simulink model "MVS_Static_Trigger_Two_Layers_RA"  (R2024a)
settings: Solver=ode5  StartTime=0.0  StopTime=180  FixedStep=0.01  RelTol=1e-3
(part 1 of 4)
settings Model: Creator=yfeih  LastModifiedBy=Lenovo
settings OptimizationCC: ReuseModelBlockBuffer=off
settings RTWCC: GPUComputeCapability=3.5

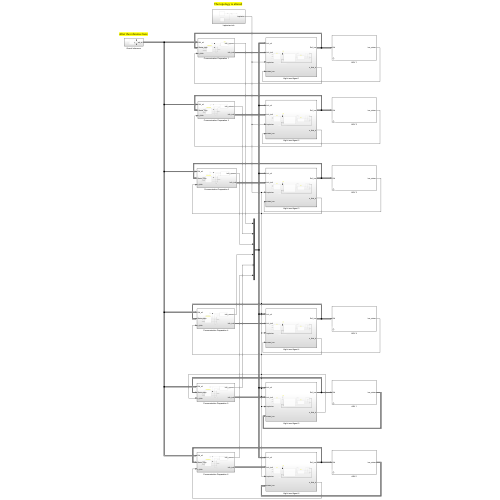
[thumbnail: Simulink's stored preview of the top-level diagram]
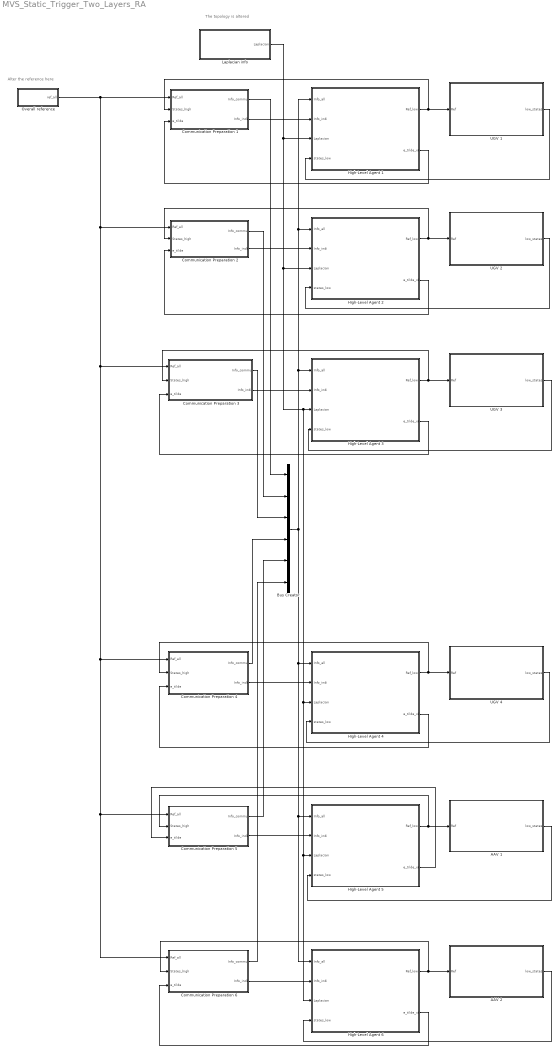
== system MVS_Static_Trigger_Two_Layers_RA ==
  note: Alter the reference here
  note: The topology is altered
  AAV 1 : Subsystem  mask{ini_pos=[-20;-20;0]}
      mask prompts: ini_pos "initial_pos"
      mask TypeOptions ini_pos: x_int/InitialCondition
      mask DialogControl ParameterGroupVar Prompt: 参数
  AAV 2 : Subsystem  mask{ini_pos=[-26;-30;0]}
      mask prompts: ini_pos "initial_pos"
      mask TypeOptions ini_pos: x_int/InitialCondition
      mask DialogControl ParameterGroupVar Prompt: 参数
  Bus Creator : BusCreator  Inputs=6
  Communication Preparation 1 : Subsystem
  Communication Preparation 2 : Subsystem
  Communication Preparation 3 : Subsystem
  Communication Preparation 4 : Subsystem
  Communication Preparation 5 : Subsystem
  Communication Preparation 6 : Subsystem
  High-Level Agent 1 : Subsystem
  High-Level Agent 2 : Subsystem
  High-Level Agent 3 : Subsystem
  High-Level Agent 4 : Subsystem
  High-Level Agent 5 : Subsystem
  High-Level Agent 6 : Subsystem
  Laplacian info : Subsystem
  Overall reference : Subsystem
  UGV 1 : Subsystem  mask{ini_int=[-25;-20;0], ini_memo=[-25;-20;0]}
      mask prompts: ini_int "initial_pos"; ini_memo "pos_memory"
      mask TypeOptions ini_int: pos_int/InitialCondition
      mask TypeOptions ini_memo: pos_memo/InitialCondition
      mask DialogControl ParameterGroupVar Prompt: 参数
  UGV 2 : Subsystem  mask{ini_int=[-35;-35;0], ini_memo=[-35;-35;0]}
      mask prompts: ini_int "initial_pos"; ini_memo "pos_memory"
      mask TypeOptions ini_int: pos_int/InitialCondition
      mask TypeOptions ini_memo: pos_memo/InitialCondition
      mask DialogControl ParameterGroupVar Prompt: 参数
  UGV 3 : Subsystem  mask{ini_int=[-50;-30;pi/4], ini_memo=[-50;-30;pi/4]}
      mask prompts: ini_int "initial_pos"; ini_memo "pos_memory"
      mask TypeOptions ini_int: pos_int/InitialCondition
      mask TypeOptions ini_memo: pos_memory/InitialCondition
      mask DialogControl ParameterGroupVar Prompt: 参数
  UGV 4 : Subsystem  mask{ini_int=[-50;-45;pi/4], ini_memo=[-50;-45;pi/4]}
      mask prompts: ini_int "initial_pos"; ini_memo "pos_memory"
      mask TypeOptions ini_int: pos_int/InitialCondition
      mask TypeOptions ini_memo: pos_memory/InitialCondition
      mask DialogControl ParameterGroupVar Prompt: 参数
  wires:
  Communication Preparation 1/1(Info_commu) -> Bus Creator/1
  Communication Preparation 1/2(Info_indi) -> High-Level Agent 1/2(Info_indi)
  High-Level Agent 1/1(Ref_low) -> UGV 1/1(Ref), Communication Preparation 1/2(States_high)
  High-Level Agent 3/1(Ref_low) -> UGV 3/1(Ref), Communication Preparation 3/2(States_high)
  Communication Preparation 3/2(Info_indi) -> High-Level Agent 3/2(Info_indi)
  Communication Preparation 3/1(Info_commu) -> Bus Creator/3
  Laplacian info/1(Laplacian) -> High-Level Agent 6/3(Laplacian), High-Level Agent 5/3(Laplacian), High-Level Agent 4/3(Laplacian), High-Level Agent 3/3(Laplacian), High-Level Agent 2/3(Laplacian), High-Level Agent 1/3(Laplacian)
  Communication Preparation 2/1(Info_commu) -> Bus Creator/2
  Communication Preparation 2/2(Info_indi) -> High-Level Agent 2/2(Info_indi)
  High-Level Agent 2/1(Ref_low) -> UGV 2/1(Ref), Communication Preparation 2/2(States_high)
  High-Level Agent 4/1(Ref_low) -> UGV 4/1(Ref), Communication Preparation 4/2(States_high)
  Communication Preparation 4/2(Info_indi) -> High-Level Agent 4/2(Info_indi)
  Communication Preparation 4/1(Info_commu) -> Bus Creator/4
  High-Level Agent 5/1(Ref_low) -> AAV 1/1(Ref), Communication Preparation 5/2(States_high)
  Communication Preparation 5/1(Info_commu) -> Bus Creator/5
  Communication Preparation 5/2(Info_indi) -> High-Level Agent 5/2(Info_indi)
  Bus Creator/1 -> High-Level Agent 6/1(Info_all), High-Level Agent 5/1(Info_all), High-Level Agent 4/1(Info_all), High-Level Agent 3/1(Info_all), High-Level Agent 2/1(Info_all), High-Level Agent 1/1(Info_all)
  High-Level Agent 6/1(Ref_low) -> AAV 2/1(Ref), Communication Preparation 6/2(States_high)
  Communication Preparation 6/1(Info_commu) -> Bus Creator/6
  Communication Preparation 6/2(Info_indi) -> High-Level Agent 6/2(Info_indi)
  Overall reference/1(ref_all) -> Communication Preparation 6/1(Ref_all), Communication Preparation 5/1(Ref_all), Communication Preparation 4/1(Ref_all), Communication Preparation 3/1(Ref_all), Communication Preparation 2/1(Ref_all), Communication Preparation 1/1(Ref_all)
  High-Level Agent 1/2(e_tilde_xi) -> Communication Preparation 1/3(e_tilde)
  High-Level Agent 2/2(e_tilde_xi) -> Communication Preparation 2/3(e_tilde)
  High-Level Agent 3/2(e_tilde_xi) -> Communication Preparation 3/3(e_tilde)
  High-Level Agent 4/2(e_tilde_xi) -> Communication Preparation 4/3(e_tilde)
  High-Level Agent 6/2(e_tilde_xi) -> Communication Preparation 6/3(e_tilde)
  High-Level Agent 5/2(e_tilde_xi) -> Communication Preparation 5/3(e_tilde)
  UGV 1/1(low_states) -> High-Level Agent 1/4(states_low)
  UGV 2/1(low_states) -> High-Level Agent 2/4(states_low)
  UGV 4/1(low_states) -> High-Level Agent 4/4(states_low)
  AAV 1/1(low_states) -> High-Level Agent 5/4(states_low)
  AAV 2/1(low_states) -> High-Level Agent 6/4(states_low)
  UGV 3/1(low_states) -> High-Level Agent 3/4(states_low)

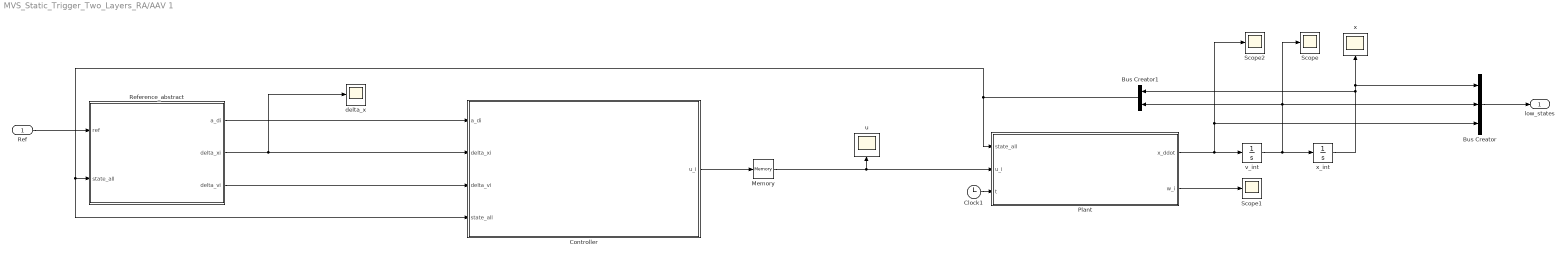
== system MVS_Static_Trigger_Two_Layers_RA/AAV 1 ==
  Ref : Inport
  Bus Creator : BusCreator  Inputs=3
  Bus Creator1 : BusCreator  Inputs=2
  Clock1 : Clock
  Controller : Subsystem
  Memory : Memory  InitialCondition=[0;0;0]
  Plant : MATLAB Function  TreatAsAtomicUnit=on
  Reference_abstract : MATLAB Function  TreatAsAtomicUnit=on
  Scope : Scope
  Scope1 : Scope
  Scope2 : Scope
  delta_x : Scope
  u : Scope
  v_int : Integrator  InitialCondition=[0;0;0]  ContinuousStateAttributes='vel'
  x : Scope
  x_int : Integrator  InitialCondition=ini_pos  ContinuousStateAttributes='pos'
  low_states : Outport
  wires:
  Plant/2(w_i) -> Scope1/1
  Clock1/1 -> Plant/3(t)
  Reference_abstract/1(a_di) -> Controller/1(a_di)
  Controller/1(u_i) -> Memory/1
  Memory/1 -> u/1, Plant/2(u_i)
  Reference_abstract/2(delta_xi) -> delta_x/1, Controller/2(delta_xi)
  Ref/1 -> Reference_abstract/1(ref)
  v_int/1 -> Bus Creator1/2, Scope/1, Bus Creator/2, x_int/1
  x_int/1 -> Bus Creator/1, x/1, Bus Creator1/1
  Reference_abstract/3(delta_vi) -> Controller/3(delta_vi)
  Bus Creator1/1 -> Controller/4(state_all), Reference_abstract/2(state_all), Plant/1(state_all)
  Bus Creator/1 -> low_states/1
  Plant/1(x_ddot) -> Scope2/1, Bus Creator/3, v_int/1

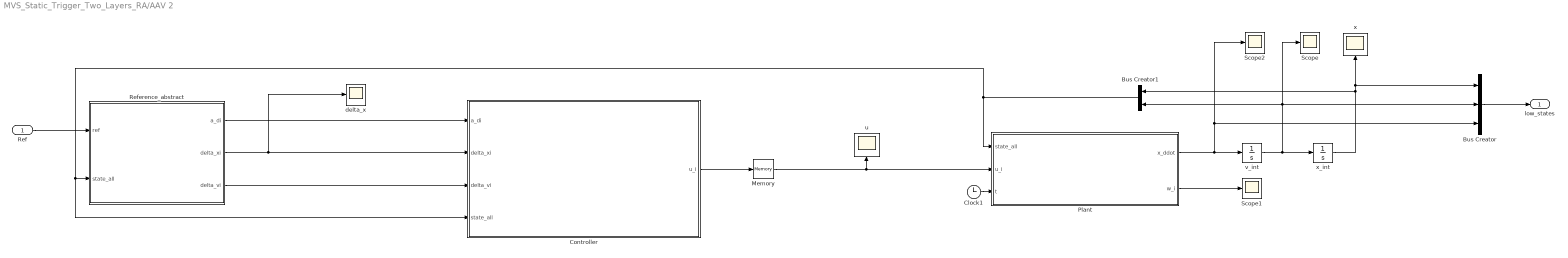
== system MVS_Static_Trigger_Two_Layers_RA/AAV 2 ==
  Ref : Inport
  Bus Creator : BusCreator  Inputs=3
  Bus Creator1 : BusCreator  Inputs=2
  Clock1 : Clock
  Controller : Subsystem
  Memory : Memory  InitialCondition=[0;0;0]
  Plant : MATLAB Function  TreatAsAtomicUnit=on
  Reference_abstract : MATLAB Function  TreatAsAtomicUnit=on
  Scope : Scope
  Scope1 : Scope
  Scope2 : Scope
  delta_x : Scope
  u : Scope
  v_int : Integrator  InitialCondition=[0;0;0]  ContinuousStateAttributes='vel'
  x : Scope
  x_int : Integrator  InitialCondition=ini_pos  ContinuousStateAttributes='pos'
  low_states : Outport
  wires:
  Plant/2(w_i) -> Scope1/1
  Clock1/1 -> Plant/3(t)
  Reference_abstract/1(a_di) -> Controller/1(a_di)
  Controller/1(u_i) -> Memory/1
  Memory/1 -> u/1, Plant/2(u_i)
  Reference_abstract/2(delta_xi) -> delta_x/1, Controller/2(delta_xi)
  Ref/1 -> Reference_abstract/1(ref)
  v_int/1 -> Bus Creator1/2, Scope/1, Bus Creator/2, x_int/1
  x_int/1 -> Bus Creator/1, x/1, Bus Creator1/1
  Reference_abstract/3(delta_vi) -> Controller/3(delta_vi)
  Bus Creator1/1 -> Controller/4(state_all), Reference_abstract/2(state_all), Plant/1(state_all)
  Bus Creator/1 -> low_states/1
  Plant/1(x_ddot) -> Scope2/1, Bus Creator/3, v_int/1

== system MVS_Static_Trigger_Two_Layers_RA/Communication Preparation 1 ==
  note: Serial number
  note: Serial number and initial position
  Ref_all : Inport
  States_high : Inport  Port=2
  e_tilde : Inport  Port=3
  Bus Creator1 : BusCreator  Inputs=3
  Event Tigger Mechanism : Subsystem
  Reference Filter : Subsystem  mask{UpperLimit=[5;5;4], LowerLimit=-[5;5;4], InitialPosition=[-25;-20;0]}
      mask prompts: UpperLimit "vel_upper_limit"; LowerLimit "vel_low_limit"; InitialPosition "initial_pos"
      mask TypeOptions UpperLimit: Speed_limit/UpperLimit
      mask TypeOptions LowerLimit: Speed_limit/LowerLimit
      mask TypeOptions InitialPosition: pos_int/InitialCondition
      mask DialogControl ParameterGroupVar Prompt: 参数
  delta_v_1 : Scope
  delta_x_1 : Scope
  Info_commu : Outport
  Info_indi : Outport  Port=2
  wires:
  Ref_all/1 -> Reference Filter/1(ref_all)
  States_high/1 -> Reference Filter/2(states_high)
  Reference Filter/1(delta_xi) -> Bus Creator1/1, Event Tigger Mechanism/1(delta_xi), delta_x_1/1
  Reference Filter/2(delta_vi) -> Event Tigger Mechanism/2(delta_vi), Bus Creator1/2, delta_v_1/1
  Reference Filter/3(acc_ref) -> Bus Creator1/3
  Bus Creator1/1 -> Info_indi/1
  Event Tigger Mechanism/1(Info_commu) -> Info_commu/1
  e_tilde/1 -> Event Tigger Mechanism/3(e_tilde)

== system MVS_Static_Trigger_Two_Layers_RA/Communication Preparation 2 ==
  note: Serial number and initial position
  Ref_all : Inport
  States_high : Inport  Port=2
  e_tilde : Inport  Port=3
  Bus Creator1 : BusCreator  Inputs=3
  Event Tigger Mechanism : Subsystem
  Reference Filter : Subsystem  mask{UpperLimit=[5;5;4], LowerLimit=-[5;5;4], InitialPosition=[-35;-35;0]}
      mask prompts: UpperLimit "vel_upper_limit"; LowerLimit "vel_low_limit"; InitialPosition "initial_pos"
      mask TypeOptions UpperLimit: Speed_limit/UpperLimit
      mask TypeOptions LowerLimit: Speed_limit/LowerLimit
      mask TypeOptions InitialPosition: pos_int/InitialCondition
      mask DialogControl ParameterGroupVar Prompt: 参数
  delta_v_2 : Scope
  delta_x_2 : Scope
  Info_commu : Outport
  Info_indi : Outport  Port=2
  wires:
  Event Tigger Mechanism/1(Info_commu) -> Info_commu/1
  Bus Creator1/1 -> Info_indi/1
  Reference Filter/3(acc_ref) -> Bus Creator1/3
  Reference Filter/2(delta_vi) -> Event Tigger Mechanism/2(delta_vi), delta_v_2/1, Bus Creator1/2
  Reference Filter/1(delta_xi) -> Bus Creator1/1, Event Tigger Mechanism/1(delta_xi), delta_x_2/1
  States_high/1 -> Reference Filter/2(states_high)
  Ref_all/1 -> Reference Filter/1(ref_all)
  e_tilde/1 -> Event Tigger Mechanism/3(e_tilde)

== system MVS_Static_Trigger_Two_Layers_RA/Communication Preparation 3 ==
  note: Serial number and initial position
  Ref_all : Inport
  States_high : Inport  Port=2
  e_tilde : Inport  Port=3
  Bus Creator1 : BusCreator  Inputs=3
  Event Tigger Mechanism : Subsystem
  Reference Filter : Subsystem  mask{UpperLimit=[5;5;4], LowerLimit=-[5;5;4], InitialPosition=[-50;-30;0]}
      mask prompts: UpperLimit "vel_upper_limit"; LowerLimit "vel_low_limit"; InitialPosition "initial_pos"
      mask TypeOptions UpperLimit: Speed_limit/UpperLimit
      mask TypeOptions LowerLimit: Speed_limit/LowerLimit
      mask TypeOptions InitialPosition: pos_int/InitialCondition
      mask DialogControl ParameterGroupVar Prompt: 参数
  delta_v_3 : Scope
  delta_x_3 : Scope
  Info_commu : Outport
  Info_indi : Outport  Port=2
  wires:
  Ref_all/1 -> Reference Filter/1(ref_all)
  States_high/1 -> Reference Filter/2(states_high)
  Reference Filter/1(delta_xi) -> Bus Creator1/1, Event Tigger Mechanism/1(delta_xi), delta_x_3/1
  Reference Filter/2(delta_vi) -> Event Tigger Mechanism/2(delta_vi), delta_v_3/1, Bus Creator1/2
  Reference Filter/3(acc_ref) -> Bus Creator1/3
  Bus Creator1/1 -> Info_indi/1
  Event Tigger Mechanism/1(Info_commu) -> Info_commu/1
  e_tilde/1 -> Event Tigger Mechanism/3(e_tilde)

== system MVS_Static_Trigger_Two_Layers_RA/Communication Preparation 4 ==
  note: Serial number and initial position
  Ref_all : Inport
  States_high : Inport  Port=2
  e_tilde : Inport  Port=3
  Bus Creator1 : BusCreator  Inputs=3
  Event Tigger Mechanism : Subsystem
  Reference Filter : Subsystem  mask{UpperLimit=[5;5;4], LowerLimit=-[5;5;4], InitialPosition=[-50;-45;0]}
      mask prompts: UpperLimit "vel_upper_limit"; LowerLimit "vel_low_limit"; InitialPosition "initial_pos"
      mask TypeOptions UpperLimit: Speed_limit/UpperLimit
      mask TypeOptions LowerLimit: Speed_limit/LowerLimit
      mask TypeOptions InitialPosition: pos_int/InitialCondition
      mask DialogControl ParameterGroupVar Prompt: 参数
  delta_v_4 : Scope
  delta_x_4 : Scope
  Info_commu : Outport
  Info_indi : Outport  Port=2
  wires:
  Ref_all/1 -> Reference Filter/1(ref_all)
  States_high/1 -> Reference Filter/2(states_high)
  Reference Filter/1(delta_xi) -> Bus Creator1/1, Event Tigger Mechanism/1(delta_xi), delta_x_4/1
  Reference Filter/2(delta_vi) -> Event Tigger Mechanism/2(delta_vi), delta_v_4/1, Bus Creator1/2
  Reference Filter/3(acc_ref) -> Bus Creator1/3
  Bus Creator1/1 -> Info_indi/1
  Event Tigger Mechanism/1(Info_commu) -> Info_commu/1
  e_tilde/1 -> Event Tigger Mechanism/3(e_tilde)

== system MVS_Static_Trigger_Two_Layers_RA/Communication Preparation 5 ==
  note: Serial number and initial position
  Ref_all : Inport
  States_high : Inport  Port=2
  e_tilde : Inport  Port=3
  Bus Creator1 : BusCreator  Inputs=3
  Event Tigger Mechanism : Subsystem
  Reference Filter : Subsystem  mask{UpperLimit=[5;5;4], LowerLimit=-[5;5;4], InitialPosition=[-20;-20;0]}
      mask prompts: UpperLimit "vel_upper_limit"; LowerLimit "vel_low_limit"; InitialPosition "initial_pos"
      mask TypeOptions UpperLimit: Speed_limit/UpperLimit
      mask TypeOptions LowerLimit: Speed_limit/LowerLimit
      mask TypeOptions InitialPosition: pos_int/InitialCondition
      mask DialogControl ParameterGroupVar Prompt: 参数
  delta_v_5 : Scope
  delta_x_5 : Scope
  Info_commu : Outport
  Info_indi : Outport  Port=2
  wires:
  Ref_all/1 -> Reference Filter/1(ref_all)
  States_high/1 -> Reference Filter/2(states_high)
  Reference Filter/1(delta_xi) -> Bus Creator1/1, Event Tigger Mechanism/1(delta_xi), delta_x_5/1
  Reference Filter/2(delta_vi) -> Event Tigger Mechanism/2(delta_vi), delta_v_5/1, Bus Creator1/2
  Reference Filter/3(acc_ref) -> Bus Creator1/3
  Bus Creator1/1 -> Info_indi/1
  Event Tigger Mechanism/1(Info_commu) -> Info_commu/1
  e_tilde/1 -> Event Tigger Mechanism/3(e_tilde)

== system MVS_Static_Trigger_Two_Layers_RA/Communication Preparation 6 ==
  note: Serial number and initial position
  Ref_all : Inport
  States_high : Inport  Port=2
  e_tilde : Inport  Port=3
  Bus Creator1 : BusCreator  Inputs=3
  Event Tigger Mechanism : Subsystem
  Reference Filter : Subsystem  mask{UpperLimit=[5;5;4], LowerLimit=-[5;5;4], InitialPosition=[-26;-30;0]}
      mask prompts: UpperLimit "vel_upper_limit"; LowerLimit "vel_low_limit"; InitialPosition "initial_pos"
      mask TypeOptions UpperLimit: Speed_limit/UpperLimit
      mask TypeOptions LowerLimit: Speed_limit/LowerLimit
      mask TypeOptions InitialPosition: pos_int/InitialCondition
      mask DialogControl ParameterGroupVar Prompt: 参数
  delta_v_6 : Scope
  delta_x_6 : Scope
  Info_commu : Outport
  Info_indi : Outport  Port=2
  wires:
  Ref_all/1 -> Reference Filter/1(ref_all)
  States_high/1 -> Reference Filter/2(states_high)
  Reference Filter/1(delta_xi) -> Bus Creator1/1, Event Tigger Mechanism/1(delta_xi), delta_x_6/1
  Reference Filter/2(delta_vi) -> Event Tigger Mechanism/2(delta_vi), delta_v_6/1, Bus Creator1/2
  Reference Filter/3(acc_ref) -> Bus Creator1/3
  Bus Creator1/1 -> Info_indi/1
  Event Tigger Mechanism/1(Info_commu) -> Info_commu/1
  e_tilde/1 -> Event Tigger Mechanism/3(e_tilde)

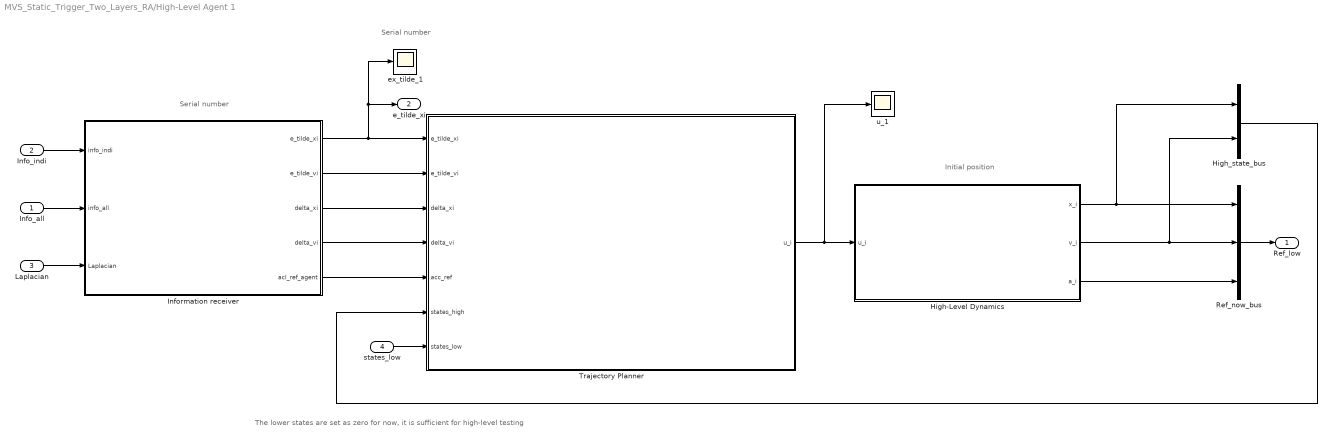
== system MVS_Static_Trigger_Two_Layers_RA/High-Level Agent 1 ==
  note: The lower states are set as zero for now, it is sufficient for high-level testing
  note: Serial number
  note: Serial number
  note: Initial position
  Info_all : Inport
  Info_indi : Inport  Port=2
  Laplacian : Inport  Port=3
  states_low : Inport  Port=4
  High-Level Dynamics : Subsystem  mask{acc_up_limit=[2;2;1.5], acc_low_limit=-[2;2;1.5], vel_up_limit=[5;5;4], vel_low_limit=-[5;5;4], ini_pos=[-25;-20;0]}
      mask prompts: ini_pos "initial_pos"
      mask TypeOptions acc_up_limit: Saturation_acc/UpperLimit
      mask TypeOptions acc_low_limit: Saturation_acc/LowerLimit
      mask TypeOptions vel_up_limit: Saturation_vel/UpperLimit
      mask TypeOptions vel_low_limit: Saturation_vel/LowerLimit
      mask TypeOptions ini_pos: Position/InitialCondition
      mask DialogControl ParameterGroupVar Prompt: 参数
  High_state_bus : BusCreator  Inputs=2
  Information receiver : MATLAB Function  TreatAsAtomicUnit=on
  Ref_now_bus : BusCreator  Inputs=3
  Trajectory Planner : Subsystem
  ex_tilde_1 : Scope
  u_1 : Scope
  Ref_low : Outport
  e_tilde_xi : Outport  Port=2
  wires:
  Info_indi/1 -> Information receiver/1(info_indi)
  Info_all/1 -> Information receiver/2(info_all)
  Laplacian/1 -> Information receiver/3(Laplacian)
  Information receiver/1(e_tilde_xi) -> e_tilde_xi/1, ex_tilde_1/1, Trajectory Planner/1(e_tilde_xi)
  Information receiver/2(e_tilde_vi) -> Trajectory Planner/2(e_tilde_vi)
  Information receiver/3(delta_xi) -> Trajectory Planner/3(delta_xi)
  Information receiver/4(delta_vi) -> Trajectory Planner/4(delta_vi)
  Information receiver/5(acl_ref_agent) -> Trajectory Planner/5(acc_ref)
  Ref_now_bus/1 -> Ref_low/1
  High-Level Dynamics/3(a_i) -> Ref_now_bus/3
  High-Level Dynamics/2(v_i) -> High_state_bus/2, Ref_now_bus/2
  High-Level Dynamics/1(x_i) -> High_state_bus/1, Ref_now_bus/1
  Trajectory Planner/1(u_i) -> u_1/1, High-Level Dynamics/1(u_i)
  High_state_bus/1 -> Trajectory Planner/6(states_high)
  states_low/1 -> Trajectory Planner/7(states_low)

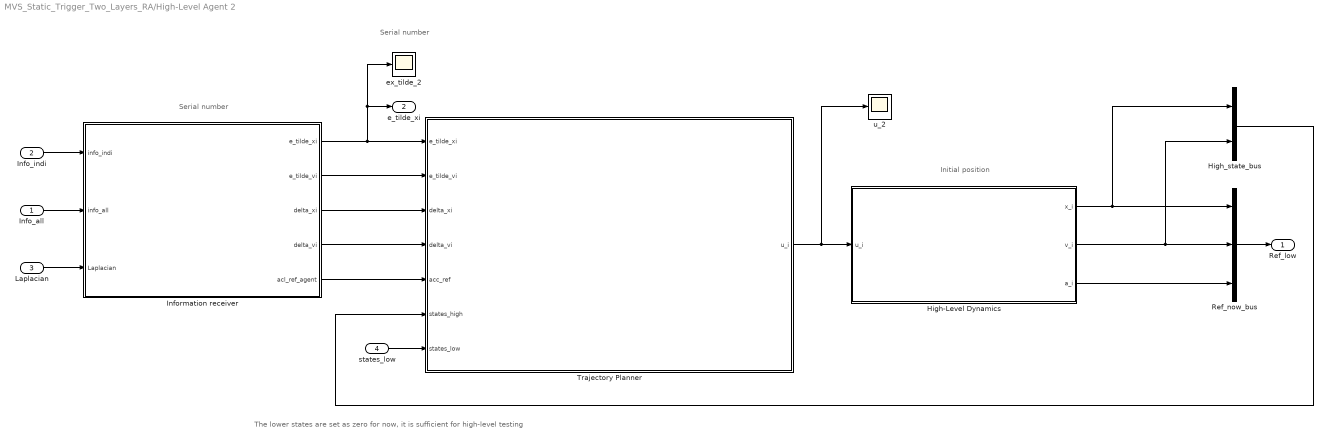
== system MVS_Static_Trigger_Two_Layers_RA/High-Level Agent 2 ==
  note: Serial number
  note: The lower states are set as zero for now, it is sufficient for high-level testing
  note: Initial position
  note: Serial number
  Info_all : Inport
  Info_indi : Inport  Port=2
  Laplacian : Inport  Port=3
  states_low : Inport  Port=4
  High-Level Dynamics : Subsystem  mask{acc_up_limit=[2;2;1.5], acc_low_limit=-[2;2;1.5], vel_up_limit=[5;5;4], vel_low_limit=-[5;5;4], ini_pos=[-35;-35;0]}
      mask prompts: ini_pos "initial_pos"
      mask TypeOptions acc_up_limit: Saturation_acc/UpperLimit
      mask TypeOptions acc_low_limit: Saturation_acc/LowerLimit
      mask TypeOptions vel_up_limit: Saturation_vel/UpperLimit
      mask TypeOptions vel_low_limit: Saturation_vel/LowerLimit
      mask TypeOptions ini_pos: Position/InitialCondition
      mask DialogControl ParameterGroupVar Prompt: 参数
  High_state_bus : BusCreator  Inputs=2
  Information receiver : MATLAB Function  TreatAsAtomicUnit=on
  Ref_now_bus : BusCreator  Inputs=3
  Trajectory Planner : Subsystem
  ex_tilde_2 : Scope
  u_2 : Scope
  Ref_low : Outport
  e_tilde_xi : Outport  Port=2
  wires:
  Info_indi/1 -> Information receiver/1(info_indi)
  Info_all/1 -> Information receiver/2(info_all)
  Laplacian/1 -> Information receiver/3(Laplacian)
  Information receiver/1(e_tilde_xi) -> ex_tilde_2/1, e_tilde_xi/1, Trajectory Planner/1(e_tilde_xi)
  Information receiver/2(e_tilde_vi) -> Trajectory Planner/2(e_tilde_vi)
  Information receiver/3(delta_xi) -> Trajectory Planner/3(delta_xi)
  Information receiver/4(delta_vi) -> Trajectory Planner/4(delta_vi)
  Information receiver/5(acl_ref_agent) -> Trajectory Planner/5(acc_ref)
  Ref_now_bus/1 -> Ref_low/1
  High-Level Dynamics/3(a_i) -> Ref_now_bus/3
  High-Level Dynamics/2(v_i) -> High_state_bus/2, Ref_now_bus/2
  High-Level Dynamics/1(x_i) -> High_state_bus/1, Ref_now_bus/1
  Trajectory Planner/1(u_i) -> u_2/1, High-Level Dynamics/1(u_i)
  High_state_bus/1 -> Trajectory Planner/6(states_high)
  states_low/1 -> Trajectory Planner/7(states_low)

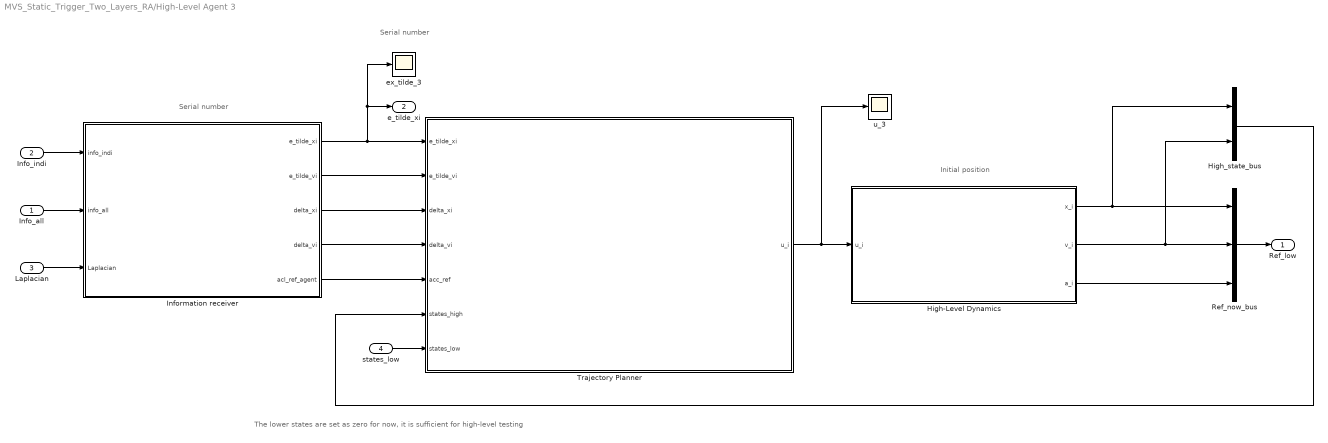
== system MVS_Static_Trigger_Two_Layers_RA/High-Level Agent 3 ==
  note: Serial number
  note: The lower states are set as zero for now, it is sufficient for high-level testing
  note: Initial position
  note: Serial number
  Info_all : Inport
  Info_indi : Inport  Port=2
  Laplacian : Inport  Port=3
  states_low : Inport  Port=4
  High-Level Dynamics : Subsystem  mask{acc_up_limit=[2;2;1.5], acc_low_limit=-[2;2;1.5], vel_up_limit=[5;5;4], vel_low_limit=-[5;5;4], ini_pos=[-50;-30;0]}
      mask prompts: ini_pos "initial_pos"
      mask TypeOptions acc_up_limit: Saturation_acc/UpperLimit
      mask TypeOptions acc_low_limit: Saturation_acc/LowerLimit
      mask TypeOptions vel_up_limit: Saturation_vel/UpperLimit
      mask TypeOptions vel_low_limit: Saturation_vel/LowerLimit
      mask TypeOptions ini_pos: Position/InitialCondition
      mask DialogControl ParameterGroupVar Prompt: 参数
  High_state_bus : BusCreator  Inputs=2
  Information receiver : MATLAB Function  TreatAsAtomicUnit=on
  Ref_now_bus : BusCreator  Inputs=3
  Trajectory Planner : Subsystem
  ex_tilde_3 : Scope
  u_3 : Scope
  Ref_low : Outport
  e_tilde_xi : Outport  Port=2
  wires:
  Info_indi/1 -> Information receiver/1(info_indi)
  Info_all/1 -> Information receiver/2(info_all)
  Laplacian/1 -> Information receiver/3(Laplacian)
  Information receiver/1(e_tilde_xi) -> e_tilde_xi/1, ex_tilde_3/1, Trajectory Planner/1(e_tilde_xi)
  Information receiver/2(e_tilde_vi) -> Trajectory Planner/2(e_tilde_vi)
  Information receiver/3(delta_xi) -> Trajectory Planner/3(delta_xi)
  Information receiver/4(delta_vi) -> Trajectory Planner/4(delta_vi)
  Information receiver/5(acl_ref_agent) -> Trajectory Planner/5(acc_ref)
  Ref_now_bus/1 -> Ref_low/1
  High-Level Dynamics/3(a_i) -> Ref_now_bus/3
  High-Level Dynamics/2(v_i) -> High_state_bus/2, Ref_now_bus/2
  High-Level Dynamics/1(x_i) -> High_state_bus/1, Ref_now_bus/1
  Trajectory Planner/1(u_i) -> u_3/1, High-Level Dynamics/1(u_i)
  High_state_bus/1 -> Trajectory Planner/6(states_high)
  states_low/1 -> Trajectory Planner/7(states_low)

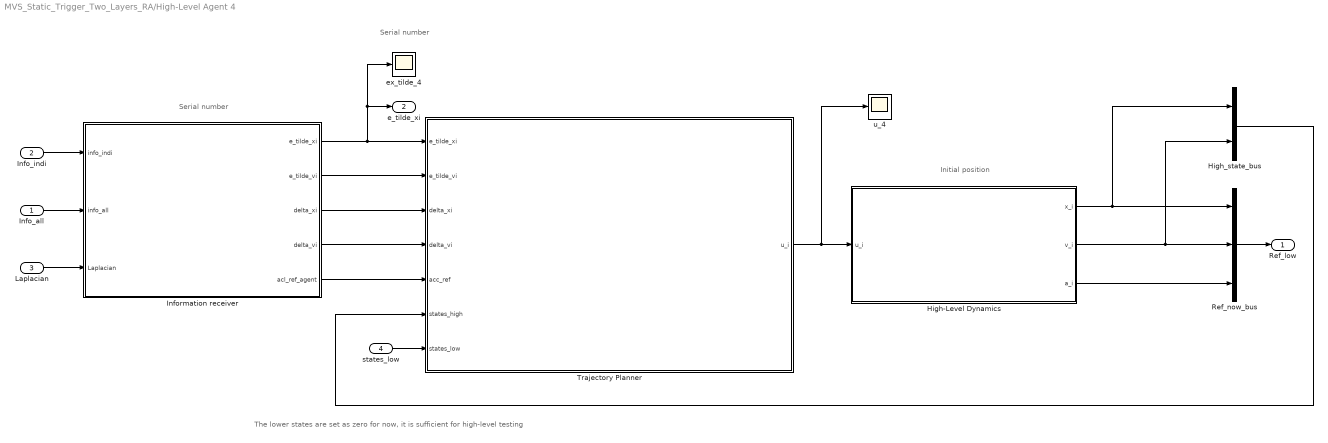
== system MVS_Static_Trigger_Two_Layers_RA/High-Level Agent 4 ==
  note: Serial number
  note: The lower states are set as zero for now, it is sufficient for high-level testing
  note: Initial position
  note: Serial number
  Info_all : Inport
  Info_indi : Inport  Port=2
  Laplacian : Inport  Port=3
  states_low : Inport  Port=4
  High-Level Dynamics : Subsystem  mask{acc_up_limit=[2;2;1.5], acc_low_limit=-[2;2;1.5], vel_up_limit=[5;5;4], vel_low_limit=-[5;5;4], ini_pos=[-50;-45;0]}
      mask prompts: ini_pos "initial_pos"
      mask TypeOptions acc_up_limit: Saturation_acc/UpperLimit
      mask TypeOptions acc_low_limit: Saturation_acc/LowerLimit
      mask TypeOptions vel_up_limit: Saturation_vel/UpperLimit
      mask TypeOptions vel_low_limit: Saturation_vel/LowerLimit
      mask TypeOptions ini_pos: Position/InitialCondition
      mask DialogControl ParameterGroupVar Prompt: 参数
  High_state_bus : BusCreator  Inputs=2
  Information receiver : MATLAB Function  TreatAsAtomicUnit=on
  Ref_now_bus : BusCreator  Inputs=3
  Trajectory Planner : Subsystem
  ex_tilde_4 : Scope
  u_4 : Scope
  Ref_low : Outport
  e_tilde_xi : Outport  Port=2
  wires:
  Info_indi/1 -> Information receiver/1(info_indi)
  Info_all/1 -> Information receiver/2(info_all)
  Laplacian/1 -> Information receiver/3(Laplacian)
  Information receiver/1(e_tilde_xi) -> ex_tilde_4/1, e_tilde_xi/1, Trajectory Planner/1(e_tilde_xi)
  Information receiver/2(e_tilde_vi) -> Trajectory Planner/2(e_tilde_vi)
  Information receiver/3(delta_xi) -> Trajectory Planner/3(delta_xi)
  Information receiver/4(delta_vi) -> Trajectory Planner/4(delta_vi)
  Information receiver/5(acl_ref_agent) -> Trajectory Planner/5(acc_ref)
  Ref_now_bus/1 -> Ref_low/1
  High-Level Dynamics/3(a_i) -> Ref_now_bus/3
  High-Level Dynamics/2(v_i) -> High_state_bus/2, Ref_now_bus/2
  High-Level Dynamics/1(x_i) -> High_state_bus/1, Ref_now_bus/1
  Trajectory Planner/1(u_i) -> u_4/1, High-Level Dynamics/1(u_i)
  High_state_bus/1 -> Trajectory Planner/6(states_high)
  states_low/1 -> Trajectory Planner/7(states_low)

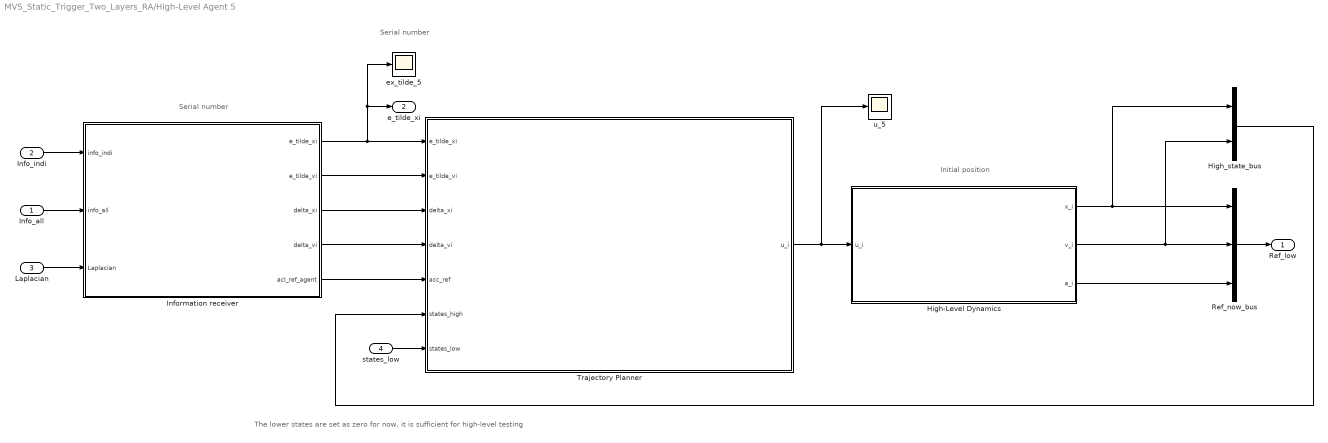
== system MVS_Static_Trigger_Two_Layers_RA/High-Level Agent 5 ==
  note: Serial number
  note: The lower states are set as zero for now, it is sufficient for high-level testing
  note: Initial position
  note: Serial number
  Info_all : Inport
  Info_indi : Inport  Port=2
  Laplacian : Inport  Port=3
  states_low : Inport  Port=4
  High-Level Dynamics : Subsystem  mask{acc_up_limit=[2;2;1.5], acc_low_limit=-[2;2;1.5], vel_up_limit=[5;5;4], vel_low_limit=-[5;5;4], ini_pos=[-20;-20;0]}
      mask prompts: ini_pos "initial_pos"
      mask TypeOptions acc_up_limit: Saturation_acc/UpperLimit
      mask TypeOptions acc_low_limit: Saturation_acc/LowerLimit
      mask TypeOptions vel_up_limit: Saturation_vel/UpperLimit
      mask TypeOptions vel_low_limit: Saturation_vel/LowerLimit
      mask TypeOptions ini_pos: Position/InitialCondition
      mask DialogControl ParameterGroupVar Prompt: 参数
  High_state_bus : BusCreator  Inputs=2
  Information receiver : MATLAB Function  TreatAsAtomicUnit=on
  Ref_now_bus : BusCreator  Inputs=3
  Trajectory Planner : Subsystem
  ex_tilde_5 : Scope
  u_5 : Scope
  Ref_low : Outport
  e_tilde_xi : Outport  Port=2
  wires:
  Info_indi/1 -> Information receiver/1(info_indi)
  Info_all/1 -> Information receiver/2(info_all)
  Laplacian/1 -> Information receiver/3(Laplacian)
  Information receiver/1(e_tilde_xi) -> e_tilde_xi/1, ex_tilde_5/1, Trajectory Planner/1(e_tilde_xi)
  Information receiver/2(e_tilde_vi) -> Trajectory Planner/2(e_tilde_vi)
  Information receiver/3(delta_xi) -> Trajectory Planner/3(delta_xi)
  Information receiver/4(delta_vi) -> Trajectory Planner/4(delta_vi)
  Information receiver/5(acl_ref_agent) -> Trajectory Planner/5(acc_ref)
  Ref_now_bus/1 -> Ref_low/1
  High-Level Dynamics/3(a_i) -> Ref_now_bus/3
  High-Level Dynamics/2(v_i) -> High_state_bus/2, Ref_now_bus/2
  High-Level Dynamics/1(x_i) -> High_state_bus/1, Ref_now_bus/1
  Trajectory Planner/1(u_i) -> u_5/1, High-Level Dynamics/1(u_i)
  High_state_bus/1 -> Trajectory Planner/6(states_high)
  states_low/1 -> Trajectory Planner/7(states_low)

== system MVS_Static_Trigger_Two_Layers_RA/High-Level Agent 6 ==
  note: Serial number
  note: The lower states are set as zero for now, it is sufficient for high-level testing
  note: Initial position
  note: Serial number
  Info_all : Inport
  Info_indi : Inport  Port=2
  Laplacian : Inport  Port=3
  states_low : Inport  Port=4
  High-Level Dynamics : Subsystem  mask{acc_up_limit=[2;2;1.5], acc_low_limit=-[2;2;1.5], vel_up_limit=[5;5;4], vel_low_limit=-[5;5;4], ini_pos=[-26;-30;0]}
      mask prompts: ini_pos "initial_pos"
      mask TypeOptions acc_up_limit: Saturation_acc/UpperLimit
      mask TypeOptions acc_low_limit: Saturation_acc/LowerLimit
      mask TypeOptions vel_up_limit: Saturation_vel/UpperLimit
      mask TypeOptions vel_low_limit: Saturation_vel/LowerLimit
      mask TypeOptions ini_pos: Position/InitialCondition
      mask DialogControl ParameterGroupVar Prompt: 参数
  High_state_bus : BusCreator  Inputs=2
  Information receiver : MATLAB Function  TreatAsAtomicUnit=on
  Ref_now_bus : BusCreator  Inputs=3
  Trajectory Planner : Subsystem
  ex_tilde_6 : Scope
  u_6 : Scope
  Ref_low : Outport
  e_tilde_xi : Outport  Port=2
  wires:
  Info_indi/1 -> Information receiver/1(info_indi)
  Info_all/1 -> Information receiver/2(info_all)
  Laplacian/1 -> Information receiver/3(Laplacian)
  Information receiver/1(e_tilde_xi) -> ex_tilde_6/1, e_tilde_xi/1, Trajectory Planner/1(e_tilde_xi)
  Information receiver/2(e_tilde_vi) -> Trajectory Planner/2(e_tilde_vi)
  Information receiver/3(delta_xi) -> Trajectory Planner/3(delta_xi)
  Information receiver/4(delta_vi) -> Trajectory Planner/4(delta_vi)
  Information receiver/5(acl_ref_agent) -> Trajectory Planner/5(acc_ref)
  Ref_now_bus/1 -> Ref_low/1
  High-Level Dynamics/3(a_i) -> Ref_now_bus/3
  High-Level Dynamics/2(v_i) -> High_state_bus/2, Ref_now_bus/2
  High-Level Dynamics/1(x_i) -> High_state_bus/1, Ref_now_bus/1
  Trajectory Planner/1(u_i) -> u_6/1, High-Level Dynamics/1(u_i)
  High_state_bus/1 -> Trajectory Planner/6(states_high)
  states_low/1 -> Trajectory Planner/7(states_low)

== system MVS_Static_Trigger_Two_Layers_RA/Laplacian info ==
  Add : Sum
  Communication topology : MATLAB Function  TreatAsAtomicUnit=on
  Constant : Constant  Value=diag(ones(6,1))  VectorParams1D=off
  Multiply : Gain  Gain=0.2
  Laplacian : Outport
  wires:
  Constant/1 -> Multiply/1
  Multiply/1 -> Add/1
  Add/1 -> Laplacian/1
  Communication topology/1(L) -> Add/2

== system MVS_Static_Trigger_Two_Layers_RA/Overall reference ==
  Bus Creator : BusCreator  Inputs=3
  Ref_gene : MATLAB Function  TreatAsAtomicUnit=on
  Time : Clock
  acc_ref : Scope
  pos_ref : Scope
  vel_ref : Scope
  ref_all : Outport
  wires:
  Bus Creator/1 -> ref_all/1
  Time/1 -> Ref_gene/1(t)
  Ref_gene/1(pos_ref) -> pos_ref/1, Bus Creator/1
  Ref_gene/3(acc_ref) -> Bus Creator/3, acc_ref/1
  Ref_gene/2(vel_ref) -> Bus Creator/2, vel_ref/1

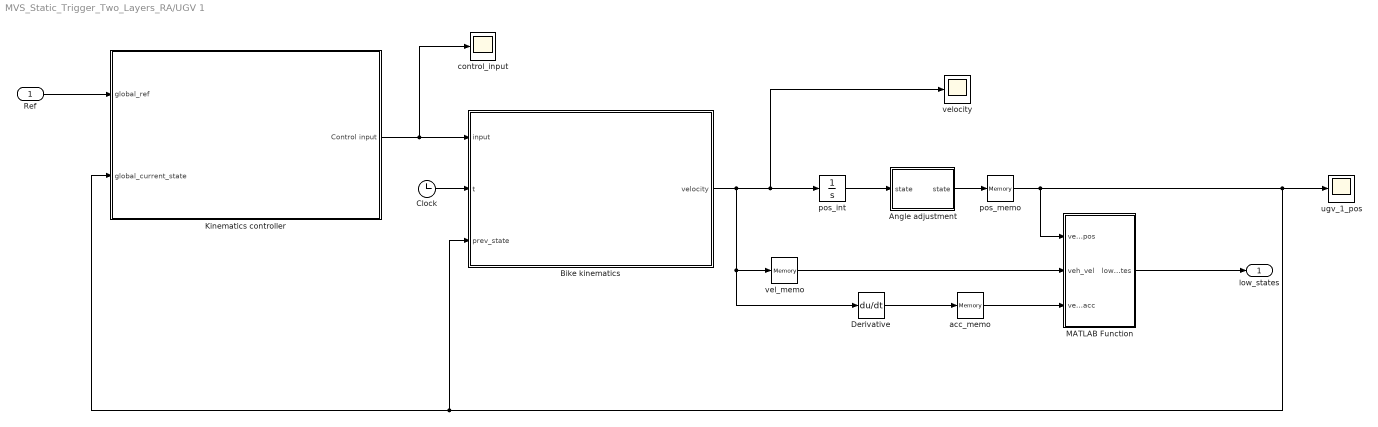
== system MVS_Static_Trigger_Two_Layers_RA/UGV 1 ==
  Ref : Inport
  Angle adjustment : MATLAB Function  TreatAsAtomicUnit=on
  Bike kinematics : MATLAB Function  TreatAsAtomicUnit=on
  Clock : Clock
  Derivative : Derivative
  Kinematics controller : Subsystem
  MATLAB Function : MATLAB Function  TreatAsAtomicUnit=on
  acc_memo : Memory  InitialCondition=zeros(3,1)
  control_input : Scope
  pos_int : Integrator  InitialCondition=ini_int
  pos_memo : Memory  InitialCondition=ini_memo
  ugv_1_pos : Scope
  vel_memo : Memory  InitialCondition=zeros(3,1)
  velocity : Scope
  low_states : Outport
  wires:
  Bike kinematics/1(velocity) -> vel_memo/1, Derivative/1, pos_int/1, velocity/1
  Angle adjustment/1(state) -> pos_memo/1
  Kinematics controller/1(Control input) -> control_input/1, Bike kinematics/1(input)
  pos_int/1 -> Angle adjustment/1("state ")
  Ref/1 -> Kinematics controller/1(global_ref)
  Derivative/1 -> acc_memo/1
  pos_memo/1 -> MATLAB Function/1(veh_pos), Bike kinematics/3(prev_state), Kinematics controller/2(global_current_state), ugv_1_pos/1
  MATLAB Function/1(low_states) -> low_states/1
  Clock/1 -> Bike kinematics/2(t)
  vel_memo/1 -> MATLAB Function/2(veh_vel)
  acc_memo/1 -> MATLAB Function/3(veh_acc)

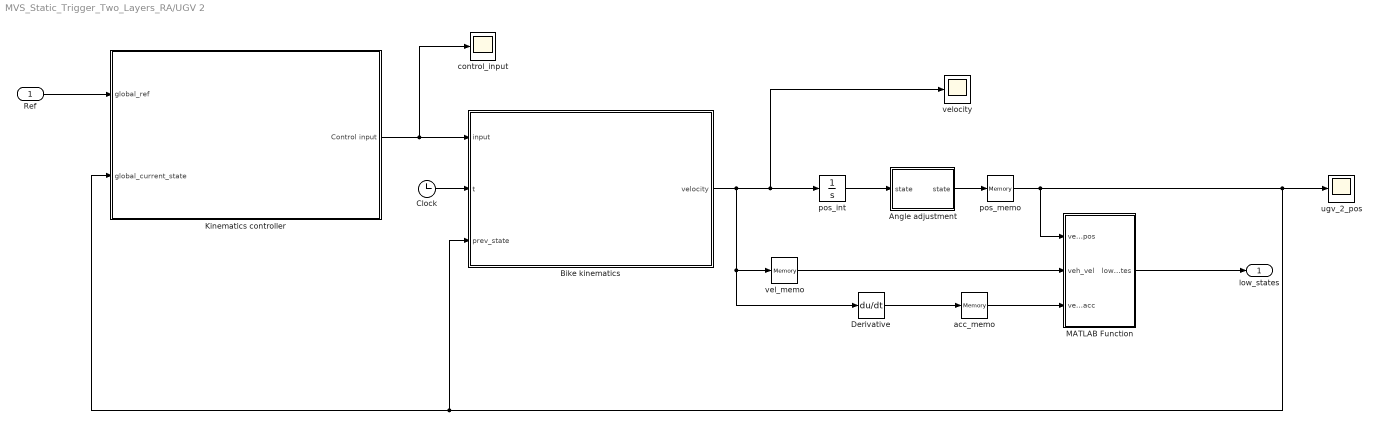
== system MVS_Static_Trigger_Two_Layers_RA/UGV 2 ==
  Ref : Inport
  Angle adjustment : MATLAB Function  TreatAsAtomicUnit=on
  Bike kinematics : MATLAB Function  TreatAsAtomicUnit=on
  Clock : Clock
  Derivative : Derivative
  Kinematics controller : Subsystem
  MATLAB Function : MATLAB Function  TreatAsAtomicUnit=on
  acc_memo : Memory  InitialCondition=zeros(3,1)
  control_input : Scope
  pos_int : Integrator  InitialCondition=ini_int
  pos_memo : Memory  InitialCondition=ini_memo
  ugv_2_pos : Scope
  vel_memo : Memory  InitialCondition=zeros(3,1)
  velocity : Scope
  low_states : Outport
  wires:
  Bike kinematics/1(velocity) -> vel_memo/1, Derivative/1, pos_int/1, velocity/1
  Angle adjustment/1(state) -> pos_memo/1
  Kinematics controller/1(Control input) -> control_input/1, Bike kinematics/1(input)
  pos_int/1 -> Angle adjustment/1("state ")
  Ref/1 -> Kinematics controller/1(global_ref)
  Derivative/1 -> acc_memo/1
  pos_memo/1 -> MATLAB Function/1(veh_pos), Bike kinematics/3(prev_state), Kinematics controller/2(global_current_state), ugv_2_pos/1
  MATLAB Function/1(low_states) -> low_states/1
  Clock/1 -> Bike kinematics/2(t)
  vel_memo/1 -> MATLAB Function/2(veh_vel)
  acc_memo/1 -> MATLAB Function/3(veh_acc)

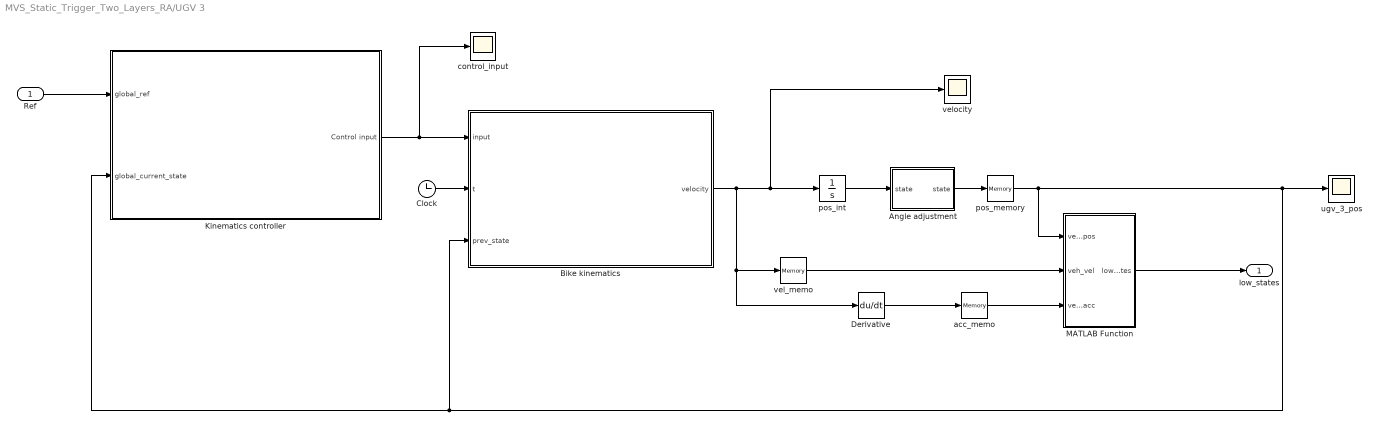
== system MVS_Static_Trigger_Two_Layers_RA/UGV 3 ==
  Ref : Inport
  Angle adjustment : MATLAB Function  TreatAsAtomicUnit=on
  Bike kinematics : MATLAB Function  TreatAsAtomicUnit=on
  Clock : Clock
  Derivative : Derivative
  Kinematics controller : Subsystem
  MATLAB Function : MATLAB Function  TreatAsAtomicUnit=on
  acc_memo : Memory  InitialCondition=zeros(3,1)
  control_input : Scope
  pos_int : Integrator  InitialCondition=ini_int
  pos_memory : Memory  InitialCondition=ini_memo
  ugv_3_pos : Scope
  vel_memo : Memory  InitialCondition=zeros(3,1)
  velocity : Scope
  low_states : Outport
  wires:
  Bike kinematics/1(velocity) -> vel_memo/1, Derivative/1, pos_int/1, velocity/1
  Angle adjustment/1(state) -> pos_memory/1
  Kinematics controller/1(Control input) -> control_input/1, Bike kinematics/1(input)
  pos_int/1 -> Angle adjustment/1("state ")
  Ref/1 -> Kinematics controller/1(global_ref)
  Derivative/1 -> acc_memo/1
  pos_memory/1 -> MATLAB Function/1(veh_pos), Bike kinematics/3(prev_state), Kinematics controller/2(global_current_state), ugv_3_pos/1
  MATLAB Function/1(low_states) -> low_states/1
  Clock/1 -> Bike kinematics/2(t)
  vel_memo/1 -> MATLAB Function/2(veh_vel)
  acc_memo/1 -> MATLAB Function/3(veh_acc)

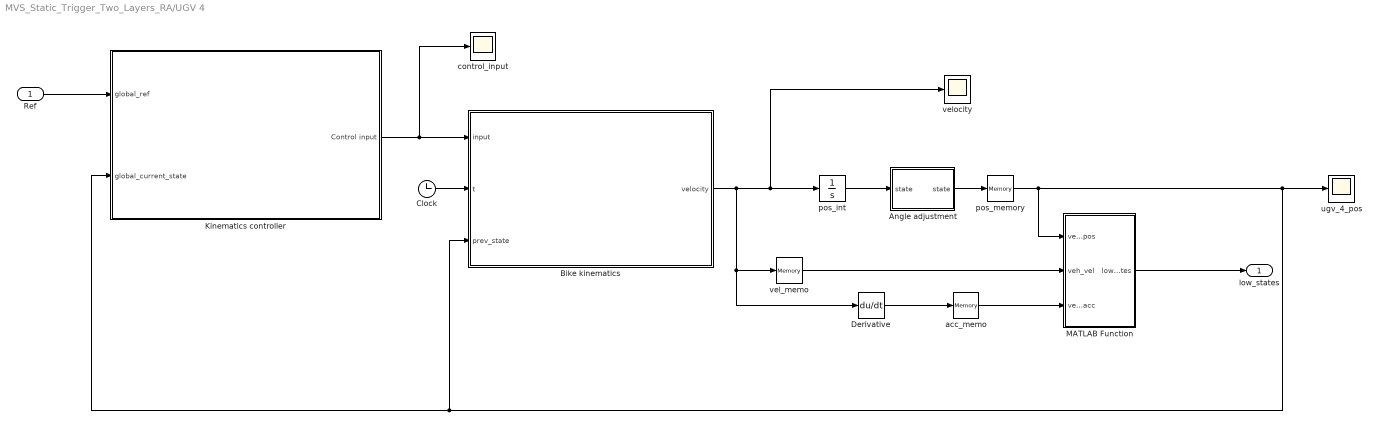
== system MVS_Static_Trigger_Two_Layers_RA/UGV 4 ==
  Ref : Inport
  Angle adjustment : MATLAB Function  TreatAsAtomicUnit=on
  Bike kinematics : MATLAB Function  TreatAsAtomicUnit=on
  Clock : Clock
  Derivative : Derivative
  Kinematics controller : Subsystem
  MATLAB Function : MATLAB Function  TreatAsAtomicUnit=on
  acc_memo : Memory  InitialCondition=zeros(3,1)
  control_input : Scope
  pos_int : Integrator  InitialCondition=ini_int
  pos_memory : Memory  InitialCondition=ini_memo
  ugv_4_pos : Scope
  vel_memo : Memory  InitialCondition=zeros(3,1)
  velocity : Scope
  low_states : Outport
  wires:
  Bike kinematics/1(velocity) -> vel_memo/1, Derivative/1, pos_int/1, velocity/1
  Angle adjustment/1(state) -> pos_memory/1
  Kinematics controller/1(Control input) -> control_input/1, Bike kinematics/1(input)
  pos_int/1 -> Angle adjustment/1("state ")
  Ref/1 -> Kinematics controller/1(global_ref)
  Derivative/1 -> acc_memo/1
  pos_memory/1 -> MATLAB Function/1(veh_pos), Bike kinematics/3(prev_state), Kinematics controller/2(global_current_state), ugv_4_pos/1
  MATLAB Function/1(low_states) -> low_states/1
  Clock/1 -> Bike kinematics/2(t)
  vel_memo/1 -> MATLAB Function/2(veh_vel)
  acc_memo/1 -> MATLAB Function/3(veh_acc)

== system MVS_Static_Trigger_Two_Layers_RA/AAV 1/Controller ==
  a_di : Inport
  delta_xi : Inport  Port=2
  delta_vi : Inport  Port=3
  state_all : Inport  Port=4
  Constant1 : Constant  Value=[0;0;0]  VectorParams1D=off
  MATLAB Function : MATLAB Function  TreatAsAtomicUnit=on
  Saturation : Saturate  UpperLimit=[2;2;12.81]  LowerLimit=[-2;-2;6.81]
  Scope : Scope
  controller : MATLAB Function  TreatAsAtomicUnit=on
  u_i : Outport
  wires:
  state_all/1 -> controller/1(state_all)
  a_di/1 -> controller/2(a_di)
  delta_xi/1 -> controller/3(delta_xi)
  controller/1(u_nom) -> MATLAB Function/1(u_nom), Saturation/1
  Constant1/1 -> controller/5(w_hat)
  delta_vi/1 -> controller/4(delta_vi)
  Saturation/1 -> MATLAB Function/2(u_sat), u_i/1
  MATLAB Function/1(u_diff) -> Scope/1

== system MVS_Static_Trigger_Two_Layers_RA/AAV 2/Controller ==
  a_di : Inport
  delta_xi : Inport  Port=2
  delta_vi : Inport  Port=3
  state_all : Inport  Port=4
  Constant1 : Constant  Value=[0;0;0]  VectorParams1D=off
  MATLAB Function : MATLAB Function  TreatAsAtomicUnit=on
  Saturation : Saturate  UpperLimit=[2;2;12.81]  LowerLimit=[-2;-2;6.81]
  Scope : Scope
  controller : MATLAB Function  TreatAsAtomicUnit=on
  u_i : Outport
  wires:
  state_all/1 -> controller/1(state_all)
  a_di/1 -> controller/2(a_di)
  delta_xi/1 -> controller/3(delta_xi)
  controller/1(u_nom) -> MATLAB Function/1(u_nom), Saturation/1
  Constant1/1 -> controller/5(w_hat)
  delta_vi/1 -> controller/4(delta_vi)
  Saturation/1 -> MATLAB Function/2(u_sat), u_i/1
  MATLAB Function/1(u_diff) -> Scope/1

== system MVS_Static_Trigger_Two_Layers_RA/Communication Preparation 1/Event Tigger Mechanism ==
  delta_xi : Inport
  delta_vi : Inport  Port=2
  e_tilde : Inport  Port=3
  Clock : Clock
  E_norm_1 : Scope
  Event trigger : MATLAB Function  TreatAsAtomicUnit=on
  Memory : Memory  InitialCondition=zeros(6,1)
  Memory1 : Memory  InitialCondition=1.5
  beta_h_1 : Scope
  high_flag_1 : Scope
  high_trigger_info_1 : Scope
  Info_commu : Outport
  wires:
  delta_vi/1 -> Event trigger/3(delta_vi_now)
  delta_xi/1 -> Event trigger/2(delta_xi_now)
  Event trigger/4(beta_i) -> Memory1/1
  Event trigger/2(trigger_flag) -> high_flag_1/1
  Memory1/1 -> beta_h_1/1, Event trigger/6(beta_i_prev)
  Memory/1 -> high_trigger_info_1/1, Event trigger/5(info_prev), Info_commu/1
  e_tilde/1 -> Event trigger/4(e_tilde)
  Event trigger/3(info_trigger) -> Memory/1
  Event trigger/1(E_norm) -> E_norm_1/1
  Clock/1 -> Event trigger/1(time)

== system MVS_Static_Trigger_Two_Layers_RA/Communication Preparation 1/Reference Filter ==
  note: Change the serial number here.
  ref_all : Inport
  states_high : Inport  Port=2
  Adaptive filter : Subsystem
  Communication-Receiver : MATLAB Function  TreatAsAtomicUnit=on
  Error Calculation : MATLAB Function  TreatAsAtomicUnit=on
  Speed_limit : Saturate  UpperLimit=UpperLimit  LowerLimit=LowerLimit
  high_error_1 : Scope
  pos_int : Integrator  InitialCondition=InitialPosition
  delta_xi : Outport
  delta_vi : Outport  Port=2
  acc_ref : Outport  Port=3
  wires:
  Communication-Receiver/3(acl_ref_agent) -> acc_ref/1
  ref_all/1 -> Communication-Receiver/1(ref_all)
  Speed_limit/1 -> pos_int/1, Error Calculation/1(vel_cur)
  Communication-Receiver/2(vel_ref_agent) -> Adaptive filter/2(vel_ref)
  Communication-Receiver/1(pos_ref_agent) -> Adaptive filter/1(pos_ref)
  pos_int/1 -> Adaptive filter/3(current_pos), Error Calculation/2(pos_cur)
  Adaptive filter/1(u_i) -> Speed_limit/1
  Error Calculation/1(delta_xi) -> delta_xi/1
  states_high/1 -> Error Calculation/3(states_high)
  Error Calculation/2(delta_vi) -> delta_vi/1
  Error Calculation/3(high_error) -> high_error_1/1
  Adaptive filter/2(filter_error) -> Error Calculation/4(filter_error)

== system MVS_Static_Trigger_Two_Layers_RA/Communication Preparation 2/Event Tigger Mechanism ==
  delta_xi : Inport
  delta_vi : Inport  Port=2
  e_tilde : Inport  Port=3
  Clock : Clock
  E_norm_2 : Scope
  Event trigger : MATLAB Function  TreatAsAtomicUnit=on
  Memory : Memory  InitialCondition=zeros(6,1)
  Memory1 : Memory  InitialCondition=1.5
  beta_h_2 : Scope
  high_flag_2 : Scope
  high_trigger_info_2 : Scope
  Info_commu : Outport
  wires:
  delta_vi/1 -> Event trigger/3(delta_vi_now)
  delta_xi/1 -> Event trigger/2(delta_xi_now)
  Event trigger/4(beta_i) -> Memory1/1
  Event trigger/2(trigger_flag) -> high_flag_2/1
  Memory1/1 -> beta_h_2/1, Event trigger/6(beta_i_prev)
  Memory/1 -> Event trigger/5(info_prev), high_trigger_info_2/1, Info_commu/1
  e_tilde/1 -> Event trigger/4(e_tilde)
  Event trigger/3(info_trigger) -> Memory/1
  Event trigger/1(E_norm) -> E_norm_2/1
  Clock/1 -> Event trigger/1(time)

== system MVS_Static_Trigger_Two_Layers_RA/Communication Preparation 2/Reference Filter ==
  note: Change the serial number here.
  ref_all : Inport
  states_high : Inport  Port=2
  Adaptive filter : Subsystem
  Communication-Receiver : MATLAB Function  TreatAsAtomicUnit=on
  Error Calculation : MATLAB Function  TreatAsAtomicUnit=on
  Speed_limit : Saturate  UpperLimit=UpperLimit  LowerLimit=LowerLimit
  high_error_2 : Scope
  pos_int : Integrator  InitialCondition=InitialPosition
  delta_xi : Outport
  delta_vi : Outport  Port=2
  acc_ref : Outport  Port=3
  wires:
  Communication-Receiver/3(acl_ref_agent) -> acc_ref/1
  ref_all/1 -> Communication-Receiver/1(ref_all)
  Speed_limit/1 -> pos_int/1, Error Calculation/1(vel_cur)
  Communication-Receiver/2(vel_ref_agent) -> Adaptive filter/2(vel_ref)
  Communication-Receiver/1(pos_ref_agent) -> Adaptive filter/1(pos_ref)
  pos_int/1 -> Adaptive filter/3(current_pos), Error Calculation/2(pos_cur)
  Adaptive filter/1(u_i) -> Speed_limit/1
  Error Calculation/1(delta_xi) -> delta_xi/1
  states_high/1 -> Error Calculation/3(states_high)
  Error Calculation/2(delta_vi) -> delta_vi/1
  Error Calculation/3(high_error) -> high_error_2/1
  Adaptive filter/2(filter_error) -> Error Calculation/4(filter_error)

== system MVS_Static_Trigger_Two_Layers_RA/Communication Preparation 3/Event Tigger Mechanism ==
  delta_xi : Inport
  delta_vi : Inport  Port=2
  e_tilde : Inport  Port=3
  Clock : Clock
  E_norm_3 : Scope
  Event trigger : MATLAB Function  TreatAsAtomicUnit=on
  Memory : Memory  InitialCondition=zeros(6,1)
  Memory1 : Memory  InitialCondition=1.5
  beta_h_3 : Scope
  high_flag_3 : Scope
  high_trigger_info_3 : Scope
  Info_commu : Outport
  wires:
  delta_vi/1 -> Event trigger/3(delta_vi_now)
  delta_xi/1 -> Event trigger/2(delta_xi_now)
  Event trigger/4(beta_i) -> Memory1/1
  Event trigger/2(trigger_flag) -> high_flag_3/1
  Memory1/1 -> beta_h_3/1, Event trigger/6(beta_i_prev)
  Memory/1 -> Event trigger/5(info_prev), high_trigger_info_3/1, Info_commu/1
  e_tilde/1 -> Event trigger/4(e_tilde)
  Event trigger/3(info_trigger) -> Memory/1
  Event trigger/1(E_norm) -> E_norm_3/1
  Clock/1 -> Event trigger/1(time)

== system MVS_Static_Trigger_Two_Layers_RA/Communication Preparation 3/Reference Filter ==
  note: Change the serial number here.
  ref_all : Inport
  states_high : Inport  Port=2
  Adaptive filter : Subsystem
  Communication-Receiver : MATLAB Function  TreatAsAtomicUnit=on
  Error Calculation : MATLAB Function  TreatAsAtomicUnit=on
  Speed_limit : Saturate  UpperLimit=UpperLimit  LowerLimit=LowerLimit
  high_error_3 : Scope
  pos_int : Integrator  InitialCondition=InitialPosition
  delta_xi : Outport
  delta_vi : Outport  Port=2
  acc_ref : Outport  Port=3
  wires:
  Communication-Receiver/3(acl_ref_agent) -> acc_ref/1
  ref_all/1 -> Communication-Receiver/1(ref_all)
  Speed_limit/1 -> pos_int/1, Error Calculation/1(vel_cur)
  Communication-Receiver/2(vel_ref_agent) -> Adaptive filter/2(vel_ref)
  Communication-Receiver/1(pos_ref_agent) -> Adaptive filter/1(pos_ref)
  pos_int/1 -> Adaptive filter/3(current_pos), Error Calculation/2(pos_cur)
  Adaptive filter/1(u_i) -> Speed_limit/1
  Error Calculation/1(delta_xi) -> delta_xi/1
  states_high/1 -> Error Calculation/3(states_high)
  Error Calculation/2(delta_vi) -> delta_vi/1
  Error Calculation/3(high_error) -> high_error_3/1
  Adaptive filter/2(filter_error) -> Error Calculation/4(filter_error)

== system MVS_Static_Trigger_Two_Layers_RA/Communication Preparation 4/Event Tigger Mechanism ==
  delta_xi : Inport
  delta_vi : Inport  Port=2
  e_tilde : Inport  Port=3
  Clock : Clock
  E_norm_4 : Scope
  Event trigger : MATLAB Function  TreatAsAtomicUnit=on
  Memory : Memory  InitialCondition=zeros(6,1)
  Memory1 : Memory  InitialCondition=1.5
  beta_h_4 : Scope
  high_flag_4 : Scope
  high_trigger_info_4 : Scope
  Info_commu : Outport
  wires:
  delta_vi/1 -> Event trigger/3(delta_vi_now)
  delta_xi/1 -> Event trigger/2(delta_xi_now)
  Event trigger/4(beta_i) -> Memory1/1
  Event trigger/2(trigger_flag) -> high_flag_4/1
  Memory1/1 -> beta_h_4/1, Event trigger/6(beta_i_prev)
  Memory/1 -> Event trigger/5(info_prev), high_trigger_info_4/1, Info_commu/1
  e_tilde/1 -> Event trigger/4(e_tilde)
  Event trigger/3(info_trigger) -> Memory/1
  Event trigger/1(E_norm) -> E_norm_4/1
  Clock/1 -> Event trigger/1(time)

== system MVS_Static_Trigger_Two_Layers_RA/Communication Preparation 4/Reference Filter ==
  note: Change the serial number here.
  ref_all : Inport
  states_high : Inport  Port=2
  Adaptive filter : Subsystem
  Communication-Receiver : MATLAB Function  TreatAsAtomicUnit=on
  Error Calculation : MATLAB Function  TreatAsAtomicUnit=on
  Speed_limit : Saturate  UpperLimit=UpperLimit  LowerLimit=LowerLimit
  high_error_4 : Scope
  pos_int : Integrator  InitialCondition=InitialPosition
  delta_xi : Outport
  delta_vi : Outport  Port=2
  acc_ref : Outport  Port=3
  wires:
  Communication-Receiver/3(acl_ref_agent) -> acc_ref/1
  ref_all/1 -> Communication-Receiver/1(ref_all)
  Speed_limit/1 -> pos_int/1, Error Calculation/1(vel_cur)
  Communication-Receiver/2(vel_ref_agent) -> Adaptive filter/2(vel_ref)
  Communication-Receiver/1(pos_ref_agent) -> Adaptive filter/1(pos_ref)
  pos_int/1 -> Adaptive filter/3(current_pos), Error Calculation/2(pos_cur)
  Adaptive filter/1(u_i) -> Speed_limit/1
  Error Calculation/1(delta_xi) -> delta_xi/1
  states_high/1 -> Error Calculation/3(states_high)
  Error Calculation/2(delta_vi) -> delta_vi/1
  Error Calculation/3(high_error) -> high_error_4/1
  Adaptive filter/2(filter_error) -> Error Calculation/4(filter_error)

== system MVS_Static_Trigger_Two_Layers_RA/Communication Preparation 5/Event Tigger Mechanism ==
  delta_xi : Inport
  delta_vi : Inport  Port=2
  e_tilde : Inport  Port=3
  Clock : Clock
  E_norm_5 : Scope
  Event trigger : MATLAB Function  TreatAsAtomicUnit=on
  Memory : Memory  InitialCondition=zeros(6,1)
  Memory1 : Memory  InitialCondition=1.5
  beta_h_5 : Scope
  high_flag_5 : Scope
  high_trigger_info_5 : Scope
  Info_commu : Outport
  wires:
  delta_vi/1 -> Event trigger/3(delta_vi_now)
  delta_xi/1 -> Event trigger/2(delta_xi_now)
  Event trigger/4(beta_i) -> Memory1/1
  Event trigger/2(trigger_flag) -> high_flag_5/1
  Event trigger/3(info_trigger) -> Memory/1
  Memory1/1 -> Event trigger/6(beta_i_prev), beta_h_5/1
  Memory/1 -> Event trigger/5(info_prev), Info_commu/1, high_trigger_info_5/1
  e_tilde/1 -> Event trigger/4(e_tilde)
  Event trigger/1(E_norm) -> E_norm_5/1
  Clock/1 -> Event trigger/1(time)

== system MVS_Static_Trigger_Two_Layers_RA/Communication Preparation 5/Reference Filter ==
  note: Change the serial number here.
  ref_all : Inport
  states_high : Inport  Port=2
  Adaptive filter : Subsystem
  Communication-Receiver : MATLAB Function  TreatAsAtomicUnit=on
  Error Calculation : MATLAB Function  TreatAsAtomicUnit=on
  Speed_limit : Saturate  UpperLimit=UpperLimit  LowerLimit=LowerLimit
  high_error_5 : Scope
  pos_int : Integrator  InitialCondition=InitialPosition
  delta_xi : Outport
  delta_vi : Outport  Port=2
  acc_ref : Outport  Port=3
  wires:
  Communication-Receiver/3(acl_ref_agent) -> acc_ref/1
  ref_all/1 -> Communication-Receiver/1(ref_all)
  Speed_limit/1 -> pos_int/1, Error Calculation/1(vel_cur)
  Communication-Receiver/2(vel_ref_agent) -> Adaptive filter/2(vel_ref)
  Communication-Receiver/1(pos_ref_agent) -> Adaptive filter/1(pos_ref)
  pos_int/1 -> Adaptive filter/3(current_pos), Error Calculation/2(pos_cur)
  Adaptive filter/1(u_i) -> Speed_limit/1
  Error Calculation/1(delta_xi) -> delta_xi/1
  states_high/1 -> Error Calculation/3(states_high)
  Error Calculation/2(delta_vi) -> delta_vi/1
  Error Calculation/3(high_error) -> high_error_5/1
  Adaptive filter/2(filter_error) -> Error Calculation/4(filter_error)

== system MVS_Static_Trigger_Two_Layers_RA/Communication Preparation 6/Event Tigger Mechanism ==
  delta_xi : Inport
  delta_vi : Inport  Port=2
  e_tilde : Inport  Port=3
  Clock : Clock
  E_norm_6 : Scope
  Event trigger : MATLAB Function  TreatAsAtomicUnit=on
  Memory : Memory  InitialCondition=zeros(6,1)
  Memory1 : Memory  InitialCondition=1.5
  beta_h_6 : Scope
  high_flag_6 : Scope
  high_trigger_info_6 : Scope
  Info_commu : Outport
  wires:
  delta_vi/1 -> Event trigger/3(delta_vi_now)
  delta_xi/1 -> Event trigger/2(delta_xi_now)
  Event trigger/4(beta_i) -> Memory1/1
  Event trigger/2(trigger_flag) -> high_flag_6/1
  Event trigger/3(info_trigger) -> Memory/1
  Memory1/1 -> beta_h_6/1, Event trigger/6(beta_i_prev)
  Memory/1 -> high_trigger_info_6/1, Info_commu/1, Event trigger/5(info_prev)
  e_tilde/1 -> Event trigger/4(e_tilde)
  Event trigger/1(E_norm) -> E_norm_6/1
  Clock/1 -> Event trigger/1(time)

== system MVS_Static_Trigger_Two_Layers_RA/Communication Preparation 6/Reference Filter ==
  note: Change the serial number here.
  ref_all : Inport
  states_high : Inport  Port=2
  Adaptive filter : Subsystem
  Communication-Receiver : MATLAB Function  TreatAsAtomicUnit=on
  Error Calculation : MATLAB Function  TreatAsAtomicUnit=on
  Speed_limit : Saturate  UpperLimit=UpperLimit  LowerLimit=LowerLimit
  high_error_6 : Scope
  pos_int : Integrator  InitialCondition=InitialPosition
  delta_xi : Outport
  delta_vi : Outport  Port=2
  acc_ref : Outport  Port=3
  wires:
  Communication-Receiver/3(acl_ref_agent) -> acc_ref/1
  ref_all/1 -> Communication-Receiver/1(ref_all)
  Speed_limit/1 -> pos_int/1, Error Calculation/1(vel_cur)
  Communication-Receiver/2(vel_ref_agent) -> Adaptive filter/2(vel_ref)
  Communication-Receiver/1(pos_ref_agent) -> Adaptive filter/1(pos_ref)
  pos_int/1 -> Adaptive filter/3(current_pos), Error Calculation/2(pos_cur)
  Adaptive filter/1(u_i) -> Speed_limit/1
  Error Calculation/1(delta_xi) -> delta_xi/1
  states_high/1 -> Error Calculation/3(states_high)
  Error Calculation/2(delta_vi) -> delta_vi/1
  Error Calculation/3(high_error) -> high_error_6/1
  Adaptive filter/2(filter_error) -> Error Calculation/4(filter_error)

== system MVS_Static_Trigger_Two_Layers_RA/High-Level Agent 1/High-Level Dynamics ==
  u_i : Inport
  Memory : Memory  InitialCondition=zeros(3,1)
  Position : Integrator  InitialCondition=ini_pos
  Saturation_acc : Saturate  UpperLimit=acc_up_limit  LowerLimit=acc_low_limit
  Saturation_vel : Saturate  UpperLimit=vel_up_limit  LowerLimit=vel_low_limit
  Speed : Integrator  InitialCondition=[0;0;0]
  v_1 : Scope
  x_1 : Scope
  x_i : Outport
  v_i : Outport  Port=2
  a_i : Outport  Port=3
  wires:
  Position/1 -> x_i/1, x_1/1
  u_i/1 -> Memory/1
  Saturation_acc/1 -> a_i/1, Speed/1
  Speed/1 -> v_1/1, Saturation_vel/1
  Saturation_vel/1 -> v_i/1, Position/1
  Memory/1 -> Saturation_acc/1
